simulink model "c9mdde3"  (R2019b)
settings: Solver=ode15s  StartTime=0.0  StopTime=1  FixedStep=0.001  RelTol=1e-10  AbsTol=eps  EnableMultiTasking=on
PreLoadFcn:
  | ww=[1e-5 1e5]; N=20;
  | a=-1;
model workspace (MAT data in the model file):
  Kd = 0.915824952486
  Ki = 0.421761282626
  Kp = 0.141886338627
  a = -0.999986491186
libraries: cstblocks x2
settings Model: Creator=toshiba  LastModifiedBy=xuedi
settings SolverCC: MaxConsecutiveMinStep=100
settings DataIOCC: MaxDataPoints=10000  SaveFormat=Array  SignalLoggingSaveFormat=ModelDataLogs  ReturnWorkspaceOutputs=off
settings OptimizationCC: ExpressionDepthLimit=2147483647  LifeSpan=inf
settings DebuggingCC: UnderspecifiedInitializationDetection=Classic  MergeDetectMultiDrivingBlocksExec=none  FcnCallInpInsideContextMsg=warning  StateNameClashWarn=warning  SFUnexpectedBacktrackingDiag=warning  SFNoUnconditionalDefaultTransitionDiag=warning  SFExecutionAtInitializationDiag=none  ArithmeticOperatorsInVariantConditions=warning
settings HardwareCC: ProdBitPerPointer=32  ProdBitPerSizeT=32  ProdBitPerPtrDiffT=32  ProdLargestAtomicFloat=None  ProdIntDivRoundTo=Undefined  ProdEndianess=Unspecified  ProdWordSize=32  ProdHWDeviceType=32-bit Generic
settings ModelReferenceCC: PropagateSignalLabelsOutOfModel=off
settings SFSimCC: SimUseLocalCustomCode=off  CustomCodeUndefinedFunction=UseInterfaceOnly
settings RTWCC: RTWUseLocalCustomCode=off
settings CodeAppCC: StateflowObjectComments=on
settings GRTTargetCC: TargetLangStandard=C89/C90 (ANSI)  CombineOutputUpdateFcns=off  GRTInterface=on
settings ConfigComp: CovMetricSettings=dw  CovSaveCumulativeToWorkspaceVar=on  CovSaveSingleToWorkspaceVar=on  CovExternalEMLEnable=off

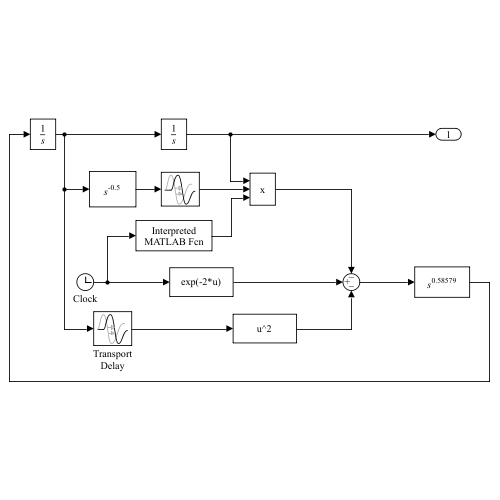
[thumbnail: Simulink's stored preview of the top-level diagram]
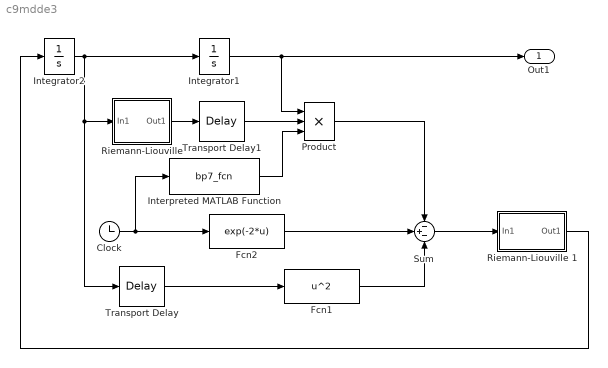
== system c9mdde3 ==
  Clock : Clock
  Fcn1 : Fcn  Expr=u^2
  Fcn2 : Fcn  Expr=exp(-2*u)
  Integrator1 : Integrator  InitialCondition=1
  Integrator2 : Integrator  InitialCondition=-1
  Interpreted MATLAB Function : MATLABFcn  MATLABFcn=bp7_fcn  Output1D=off
  Product : Product  Inputs=***  RndMeth=Zero
  "Riemann-Liouville " : Subsystem  mask{gam=-0.5, ww=ww, n=N, kF1=off, kF=Oustaloup filter}
      mask prompts: gam "Derivative order gamma"; ww "Frequency range [wb,wh]"; n "Apprixmation order"; kF1 "Is a low-pass filter required?"; kF "Filter type"
      mask init:
      | wb=ww(1); wh=ww(2); 
      | if isnumeric(gam), str=['{\its}^{' num2str(gam) '}']; 
      | else, str='{\its}^{\gamma}'; end
      | if kF==1, G=ousta_fod(gam,n,wb,wh);
      | elseif kF==2, G=new_fod(gam,n,wb,wh); 
      | else, G=matsuda_fod(gam,n,wb,wh); end
      | T=1/wh; if kF1==1, G=G*tf(1,[T 1]); end
      mask TypeOptions kF: Oustaloup filter | Modified Oustaloup filter | Matsuda-Fujii filter
      mask Display: disp(str,'texmode','on')
  Riemann-Liouville 1 : Subsystem  mask{gam=2-sqrt(2), ww=ww, n=N, kF1=off, kF=Oustaloup filter}
      mask prompts: gam "Derivative order gamma"; ww "Frequency range [wb,wh]"; n "Apprixmation order"; kF1 "Is a low-pass filter required?"; kF "Filter type"
      mask init: same as c9mdde3/Riemann-Liouville 
      mask TypeOptions kF: Oustaloup filter | Modified Oustaloup filter | Matsuda-Fujii filter
      mask Display: disp(str,'texmode','on')
  Sum : Sum  Inputs=-+-
  Transport Delay : TransportDelay  DelayTime=0.1  BufferSize=1024*4
  Transport Delay1 : TransportDelay  DelayTime=0.2  BufferSize=1024*4
  Out1 : Outport
  wires:
  Integrator1/1 -> Out1/1, Product/1
  Integrator2/1 -> Transport Delay/1, "Riemann-Liouville "/1(In1), Integrator1/1
  Fcn2/1 -> Sum/2
  Sum/1 -> Riemann-Liouville 1/1(In1)
  Riemann-Liouville 1/1(Out1) -> Integrator2/1
  "Riemann-Liouville "/1(Out1) -> Transport Delay1/1
  Product/1 -> Sum/1
  Clock/1 -> Fcn2/1, Interpreted MATLAB Function/1
  Interpreted MATLAB Function/1 -> Product/3
  Transport Delay/1 -> Fcn1/1
  Fcn1/1 -> Sum/3
  Transport Delay1/1 -> Product/2

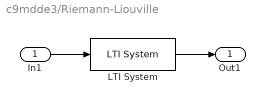
== system c9mdde3/Riemann-Liouville  ==
  In1 : Inport
  LTI System : cstblocks/LTI System  sys=G  IC=[]
  Out1 : Outport
  wires:
  LTI System/1 -> Out1/1
  In1/1 -> LTI System/1

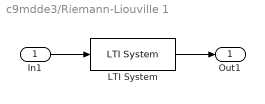
== system c9mdde3/Riemann-Liouville 1 ==
  In1 : Inport
  LTI System : cstblocks/LTI System  sys=G  IC=[]
  Out1 : Outport
  wires:
  LTI System/1 -> Out1/1
  In1/1 -> LTI System/1
